simulink model "HyQ2Max_Leg_2Dof_ForAc1"  (Simulink 7.0)
settings: Solver=ode15s  StartTime=0.0  StopTime=6.0  MaxStep=1e-2  RelTol=1e-3
values from neighbouring files (symbols this model uses):
  L_LegInertiab_CAD = [ ... (first row only)    [HyQ2Max_CAD_For_SimMechanics_LF_RF.m]
  L_LegMb = 1.406    [HyQ2Max_CAD_For_SimMechanics_LF_RF.m]
  U_LegInertia_CAD = [0.010196 0.002320 0.000141 ... (first row only)    [HyQ2Max_CAD_For_SimMechanics_LF_RF.m]
  U_LegM = 4.95    [HyQ2Max_CAD_For_SimMechanics_LF_RF.m]
libraries: mblibv1 x24, fl_lib x6, nesl_utility x4, simulink_extras x2
settings Model: Creator=Gustavo  LastModifiedBy=Gustavo
settings SolverCC: SolverResetMethod=Robust
settings DebuggingCC: SaveWithParameterizedLinksMsg=none  SignalResolutionControl=TryResolveAllWithWarning  MultiTaskDSMMsg=warning  MultiTaskCondExecSysMsg=none
settings RTWCC: IncludeERTFirstTime=on
settings GRTTargetCC: TargetFcnLib=ansi_tfl_tmw.mat
settings SimMechanicsCC: VisOnUpdateDiagram=on  VisDuringSimulation=on

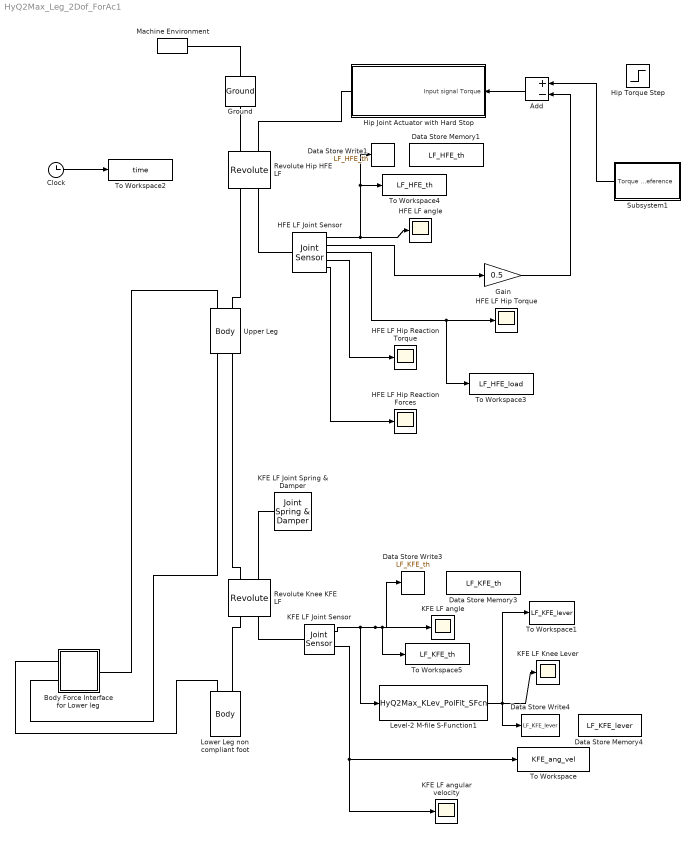
== system HyQ2Max_Leg_2Dof_ForAc1 ==
  Add : Sum  Orientation=left  Inputs=+-  OutDataType=sfix(16)  OutScaling=2^-10
  Body Force Interface for Lower leg : Subsystem
  Clock : Clock
      settings: Decimation=10
  Data Store Memory1 : DataStoreMemory  DataStoreName=LF_HFE_th  ReadBeforeWriteMsg=warning  WriteAfterWriteMsg=warning  WriteAfterReadMsg=warning  OutDataType=sfix(16)  OutScaling=2^0
  Data Store Memory3 : DataStoreMemory  DataStoreName=LF_KFE_th  ReadBeforeWriteMsg=warning  WriteAfterWriteMsg=warning  WriteAfterReadMsg=warning  OutDataType=sfix(16)  OutScaling=2^0
  Data Store Memory4 : DataStoreMemory  DataStoreName=LF_KFE_lever  ReadBeforeWriteMsg=warning  WriteAfterWriteMsg=warning  WriteAfterReadMsg=warning  OutDataType=sfix(16)  OutScaling=2^0
  Data Store Write1 : DataStoreWrite  DataStoreName=LF_HFE_th  SampleTime=-1
  Data Store Write3 : DataStoreWrite  DataStoreName=LF_KFE_th  SampleTime=-1
  Data Store Write4 : DataStoreWrite  DataStoreName=LF_KFE_lever  SampleTime=-1
  Gain : Gain  Gain=0.5  ParameterDataType=sfix(16)  ParameterScaling=2^0  OutDataType=sfix(16)  OutScaling=2^0
  Ground : mblibv1/Bodies/Ground  Orientation=down  DialogController=MECH.DynMechDlgSource  SystemSampleTime=-1  LeftPortType=env  RightPortType=workingframe  PhysicalDomain=Mechanical  DialogClass=GroundBlock  CoordPosition=[0 0 0]  CoordPositionUnits=m  StateVectorMgrId=-1  MachineId=[0 0]  ShowEnvPort=on
  HFE LF Joint Sensor : mblibv1/Sensors &  Actuators/Joint Sensor  DialogController=MECH.DynMechDlgSource  SystemSampleTime=-1  PhysicalDomain=Mechanical  PortType=blob  Muxed=off  Pose=off  Angle=on  AngleUnits=rad  ArcVelocity=on  ArcVelocityUnits=rad/s  ArcAcceleration=off  ArcAccelerationUnits=rad/s^2  CoordPosition=on  CoordPositionUnits=m  Velocity=off  VelocityUnits=m/s  Acceleration=off  AccelerationUnits=m/s^2  Quaternion=on  QuaternionDT=off  QuaternionDDT=off  QuaternionUnits=off  OutputVector=[ 1 ]  ActiveIO=on  Width=9  DialogClass=MechanicalSensorBlock  Primitive=R1  Force=off  ForceUnits=N  Torque=on  TorqueUnits=N*m  ReferenceFrame=Absolute (INERTIAL)  ReactionSensedSide=Base  ReactionReferenceFrame=Absolute (World)  ReactionForce=on  ReactionForceUnits=N  ReactionMoment=on  ReactionMomentUnits=N*m
  HFE LF Hip Reaction Forces : Scope
      settings: YMin=-40  YMax=40  SaveName=ScopeData6
  HFE LF Hip Reaction Torque : Scope
      settings: YMin=-0.4  YMax=0.3  SaveName=ScopeData7
  HFE LF Hip Torque : Scope
      settings: TimeRange=6  YMin=-10000  YMax=10000  SaveName=ScopeData4
  HFE LF angle : Scope
      settings: YMin=-0.1  YMax=1
  Hip Joint Actuator with Hard Stop : Subsystem  Orientation=left
  Hip Torque Step : Step  Orientation=left  After=5  SampleTime=0
  KFE LF Joint Sensor : mblibv1/Sensors &  Actuators/Joint Sensor  DialogController=MECH.DynMechDlgSource  SystemSampleTime=-1  PhysicalDomain=Mechanical  PortType=blob  Muxed=off  Pose=off  Angle=on  AngleUnits=rad  ArcVelocity=on  ArcVelocityUnits=rad/s  ArcAcceleration=off  ArcAccelerationUnits=rad/s^2  CoordPosition=on  CoordPositionUnits=m  Velocity=off  VelocityUnits=m/s  Acceleration=off  AccelerationUnits=m/s^2  Quaternion=on  QuaternionDT=off  QuaternionDDT=off  QuaternionUnits=off  OutputVector=[ 1 ]  ActiveIO=on  Width=2  DialogClass=MechanicalSensorBlock  Primitive=R1  Force=off  ForceUnits=N  Torque=off  TorqueUnits=N*m  ReferenceFrame=Absolute (INERTIAL)  ReactionSensedSide=Base  ReactionReferenceFrame=Absolute (World)  ReactionForce=off  ReactionForceUnits=N  ReactionMoment=off  ReactionMomentUnits=N*m
  KFE LF Joint Spring & Damper : mblibv1/Force  Elements/Joint Spring & Damper  DialogController=MECH.DynMechDlgSource  SystemSampleTime=-1  DialogClass=JointSpringDamper  JFEParameters=P1$false$0$0$0$m$m/s$N$deg$deg/s$N*m#P2$false$0$0$0$m$m/s$N$deg$deg/s$N*m#P3$false$0$0$0$m$m/s$N$deg$deg/s$N*m#R1$true$0$0.5$0$m$m/s$N$rad$rad/s$N*m#R2$false$0$0$0$m$m/s$N$deg$deg/s$N*m#R3$false$0$0$0$m$m/s$N$deg$deg/s$N*m#S$false$0$0$0$m$m/s$N$deg$deg/s$N*m
  KFE LF Knee Lever : Scope
      settings: YMin=0.005  YMax=0.04  SaveName=ScopeData9
  KFE LF angle : Scope
      settings: YMin=-2.5  YMax=0  SaveName=ScopeData8
  KFE LF angular velocity : Scope
      settings: YMin=-3.5  YMax=3.5
  Level-2 M-file S-Function1 : M-S-Function  FunctionName=HyQ2Max_KLev_PolFit_SFcn
  Lower Leg non compliant foot : mblibv1/Bodies/Body  Orientation=down  DialogController=MECH.DynMechDlgSource  PhysicalDomain=mechanical  SubClassName=Unknown  LeftPortType=workingframe  RightPortType=workingframe  LConnTagsString=CS3|CS1  RConnTagsString=CS2  DialogClass=MechanicalBodyBlock  Mass=L_LegMb  MassUnits=kg  InertiaUnits=kg*m^2  Inertia=L_LegInertiab_CAD  Shape=Cylinder  ShapeDims=[1 1]  ShapeUnits=m  ShapeUse=false  Density=1  DensityUnits=kg/m^3  DensityUse=false  CG=Left$CG$L_LegCogb_CAD$CS1$CS1$m$[-90 180 0]$Euler Z-X-Z$deg$World$false  WorkingFrames="Left$CS3$[0.0262 0.0216 0]$CS1$CS1$m$[-90 180 0]$Euler Z-X-Z$deg$World$true#Left$CS1$[0 0  0]$Adjoining$Adjoining$m$[-90 180 0]$Euler Z-X-Z$deg$World$true#Right$CS2$[0.38009 0 0]$CS1$CS1$m$[-90 180 0]$Euler Z-X-Z$deg$World$true"  CGPos=L_LegCogb_CAD  CGRot=[-90 180 0]  CS0Pos=[]  CS0Rot=[]  CS1Pos="[0 0  0]"  CS1Rot=[-90 180 0]  CS2Pos=[0.38009 0 0]  CS2Rot=[-90 180 0]  CS3Pos=[0.0262 0.0216 0]  CS3Rot=[-90 180 0]  CS4Pos=[]  CS4Rot=[]  CS5Pos=[]  CS5Rot=[]  CS6Pos=[]  CS6Rot=[]  CS7Pos=[]  CS7Rot=[]  CS8Pos=[]  CS8Rot=[]  CS9Pos=[]  CS9Rot=[]  CS10Pos=[]  CS10Rot=[]  CS11Pos=[]  CS11Rot=[]  CS12Pos=[]  CS12Rot=[]  CS13Pos=[]  CS13Rot=[]  CS14Pos=[]  CS14Rot=[]  CS15Pos=[]  CS15Rot=[]  CS16Pos=[]  CS16Rot=[]  CS17Pos=[]  CS17Rot=[]  CS18Pos=[]  CS18Rot=[]  CS19Pos=[]  CS19Rot=[]  CS20Pos=[]  CS20Rot=[]
  Machine Environment : mblibv1/Bodies/Machine Environment  Tag=Factory ground  DialogController=MECH.DialogSource  SystemSampleTime=-1  PortType=env  PhysicalDomain=Mechanical  DialogTemplateClass=MECH.MachineEnvironment  SyncWhenCopied=off  Gravity=[0 -9.81 0]  GravityUnits=m/s^2  GravityAsSignal=off  Dimensionality=Auto-detect  AnalysisType=Forward dynamics  LinearAssemblyTolerance=1e-3  LinearAssemblyToleranceUnits=m  AngularAssemblyTolerance=1e-3  AngularAssemblyToleranceUnits=rad  ConstraintSolverType=Stabilizing  ConstraintRelTolerance=1e-4  ConstraintAbsTolerance=1e-4  UseRobustSingularityHandling=off  RedundancyAnalysisToleranceType=Automatically select tolerance  RedundancyAnalysisTolerance=1e-14  StatePerturbationType=Fixed  PerturbationSize=1e-5  VisualizeMachine=on
  Revolute Hip HFE LF : mblibv1/Joints/Revolute  Orientation=down  DialogController=MECH.DynMechDlgSource  PhysicalDomain=mechanical  SubClassName=Unknown  LeftPortType=blob  RightPortType=blob  LConnTagsString=__newl0|SA1  RConnTagsString=__newr0|SA1  NumSAPorts=2  CutJoint=off  MarkAsCut=off  Primitives=revolute  PrimitiveProps=R1$World$[0 0 -1]$revolute  DialogClass=JointBlock  R1Axis=[0 0 -1]
  Revolute Knee KFE LF : mblibv1/Joints/Revolute  Orientation=down  DialogController=MECH.DynMechDlgSource  PhysicalDomain=mechanical  SubClassName=Unknown  LeftPortType=blob  RightPortType=blob  LConnTagsString=__newl0|SA1  RConnTagsString=__newr0|SA1  NumSAPorts=2  CutJoint=off  MarkAsCut=off  Primitives=revolute  PrimitiveProps=R1$World$[0 0 -1]$revolute  DialogClass=JointBlock  R1Axis=[0 0 -1]
  Subsystem1 : Subsystem  Orientation=left
  To Workspace : ToWorkspace  VariableName=KFE_ang_vel  SampleTime=-1  SaveFormat=Array
  To Workspace1 : ToWorkspace  VariableName=LF_KFE_lever  SampleTime=-1  SaveFormat=Array
  To Workspace2 : ToWorkspace  VariableName=time  SampleTime=-1  SaveFormat=Array
  To Workspace3 : ToWorkspace  VariableName=LF_HFE_load  SampleTime=-1  SaveFormat=Array
  To Workspace4 : ToWorkspace  VariableName=LF_HFE_th  SampleTime=-1  SaveFormat=Array
  To Workspace5 : ToWorkspace  VariableName=LF_KFE_th  SampleTime=-1  SaveFormat=Array
  Upper Leg : mblibv1/Bodies/Body  Orientation=down  DialogController=MECH.DynMechDlgSource  PhysicalDomain=mechanical  SubClassName=Unknown  LeftPortType=workingframe  RightPortType=workingframe  LConnTagsString=CS4|CS1  RConnTagsString=CS3|CS2  DialogClass=MechanicalBodyBlock  Mass=U_LegM  MassUnits=kg  InertiaUnits=kg*m^2  Inertia=U_LegInertia_CAD  Shape=Cylinder  ShapeDims=[1 1]  ShapeUnits=m  ShapeUse=false  Density=1  DensityUnits=kg/m^3  DensityUse=false  CG=Left$CG$U_LegCog_CAD$CS1$CS1$m$[-90 180 0]$Euler Z-X-Z$deg$WORLD$false  WorkingFrames="Left$CS4$[-.041 -.005 0]$CS1$CS1$m$[-90 180 0]$Euler Z-X-Z$deg$WORLD$true#Right$CS3$[.32  .023 0]$CS1$CS1$m$[-90 180 0]$Euler Z-X-Z$deg$WORLD$true#Left$CS1$[0 0 0]$World$World$m$[-90 180 0]$Euler Z-X-Z$deg$World$true#Right$CS2$[.36 0 0]$CS1$CS1$m$[-90 180 0]$Euler Z-X-Z$deg$World$true"  CGPos=U_LegCog_CAD  CGRot=[-90 180 0]  CS0Pos=[]  CS0Rot=[]  CS1Pos=[0 0 0]  CS1Rot=[-90 180 0]  CS2Pos=[.36 0 0]  CS2Rot=[-90 180 0]  CS3Pos="[.32  .023 0]"  CS3Rot=[-90 180 0]  CS4Pos=[-.041 -.005 0]  CS4Rot=[-90 180 0]  CS5Pos=[]  CS5Rot=[]  CS6Pos=[]  CS6Rot=[]  CS7Pos=[]  CS7Rot=[]  CS8Pos=[]  CS8Rot=[]  CS9Pos=[]  CS9Rot=[]  CS10Pos=[]  CS10Rot=[]  CS11Pos=[]  CS11Rot=[]  CS12Pos=[]  CS12Rot=[]  CS13Pos=[]  CS13Rot=[]  CS14Pos=[]  CS14Rot=[]  CS15Pos=[]  CS15Rot=[]  CS16Pos=[]  CS16Rot=[]  CS17Pos=[]  CS17Rot=[]  CS18Pos=[]  CS18Rot=[]  CS19Pos=[]  CS19Rot=[]  CS20Pos=[]  CS20Rot=[]
  wires:
  HFE LF Joint Sensor/1 -> HFE LF angle/1, To Workspace4/1, Data Store Write1/1
  KFE LF Joint Sensor/1 -> Level-2 M-file S-Function1/1, KFE LF angle/1, To Workspace5/1, Data Store Write3/1
  Level-2 M-file S-Function1/1 -> KFE LF Knee Lever/1, To Workspace1/1, Data Store Write4/1
  Gain/1 -> Add/2
  Add/1 -> Hip Joint Actuator with Hard Stop/1(Input signal Torque)
  HFE LF Joint Sensor/5 -> HFE LF Hip Reaction Forces/1
  HFE LF Joint Sensor/4 -> HFE LF Hip Reaction Torque/1
  HFE LF Joint Sensor/3 -> HFE LF Hip Torque/1, To Workspace3/1
  HFE LF Joint Sensor/2 -> Gain/1
  KFE LF Joint Sensor/2 -> KFE LF angular velocity/1, To Workspace/1
  Clock/1 -> To Workspace2/1
  Subsystem1/1(Torque Reference) -> Add/1
  connections:
  HFE LF Joint Sensor/LConn1 -- Revolute Hip HFE LF/RConn2
  Machine Environment/RConn1 -- Ground/LConn1
  Ground/RConn1 -- Revolute Hip HFE LF/LConn1
  Revolute Hip HFE LF/RConn1 -- Upper Leg/LConn2
  Upper Leg/RConn2 -- Revolute Knee KFE LF/LConn1
  KFE LF Joint Sensor/LConn1 -- Revolute Knee KFE LF/RConn2
  Lower Leg non compliant foot/LConn2 -- Revolute Knee KFE LF/RConn1
  Lower Leg non compliant foot/LConn1 -- Body Force Interface for Lower leg/LConn1
  Revolute Knee KFE LF/LConn2 -- KFE LF Joint Spring & Damper/LConn1
  Hip Joint Actuator with Hard Stop/RConn1 -- Revolute Hip HFE LF/LConn2
  Body Force Interface for Lower leg/RConn1 -- Upper Leg/LConn1
  Upper Leg/RConn1 -- Body Force Interface for Lower leg/LConn2

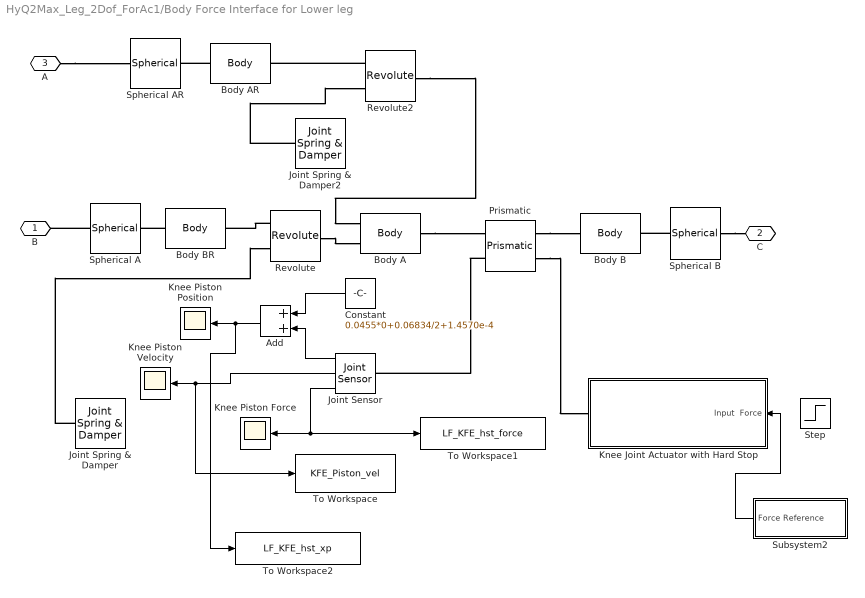
== system HyQ2Max_Leg_2Dof_ForAc1/Body Force Interface for Lower leg ==
  Add : Sum  Orientation=left  OutDataType=sfix(16)  OutScaling=2^-10
  Body A : mblibv1/Bodies/Body  DialogController=MECH.DynMechDlgSource  PhysicalDomain=mechanical  SubClassName=Unknown  LeftPortType=workingframe  RightPortType=workingframe  LConnTagsString=CS3|CS1  RConnTagsString=CS2  DialogClass=MechanicalBodyBlock  Mass=0.09  MassUnits=kg  InertiaUnits=kg*m^2  Inertia=eye(3)*1e-4  Shape=Cylinder  ShapeDims=[1 1]  ShapeUnits=m  ShapeUse=false  Density=1  DensityUnits=kg/m^3  DensityUse=false  CG=Left$CG$[-.3935857/2 0 0]$CS1$CS1$m$[0 0 0]$Euler X-Y-Z$deg$CS1$false  WorkingFrames=Left$CS3$[0 0 0]$Adjoining$Adjoining$m$[0 0 0]$Euler X-Y-Z$deg$Adjoining$true#Left$CS1$[0 0 0]$Adjoining$Adjoining$m$[0 0 -55.1441]$Euler X-Y-Z$deg$Adjoining$true#Right$CS2$[-.3935857 0 0]$CS1$CS1$m$[0 0 0]$Euler X-Y-Z$deg$CS1$true  CGPos=[-.3935857/2 0 0]  CGRot=[0 0 0]  CS0Pos=[]  CS0Rot=[]  CS1Pos=[0 0 0]  CS1Rot=[0 0 -55.1441]  CS2Pos=[-.3935857 0 0]  CS2Rot=[0 0 0]  CS3Pos=[0 0 0]  CS3Rot=[0 0 0]  CS4Pos=[]  CS4Rot=[]  CS5Pos=[]  CS5Rot=[]  CS6Pos=[]  CS6Rot=[]  CS7Pos=[]  CS7Rot=[]  CS8Pos=[]  CS8Rot=[]  CS9Pos=[]  CS9Rot=[]  CS10Pos=[]  CS10Rot=[]  CS11Pos=[]  CS11Rot=[]  CS12Pos=[]  CS12Rot=[]  CS13Pos=[]  CS13Rot=[]  CS14Pos=[]  CS14Rot=[]  CS15Pos=[]  CS15Rot=[]  CS16Pos=[]  CS16Rot=[]  CS17Pos=[]  CS17Rot=[]  CS18Pos=[]  CS18Rot=[]  CS19Pos=[]  CS19Rot=[]  CS20Pos=[]  CS20Rot=[]
  Body AR : mblibv1/Bodies/Body  DialogController=MECH.DynMechDlgSource  PhysicalDomain=mechanical  SubClassName=Unknown  LeftPortType=workingframe  RightPortType=workingframe  LConnTagsString=CS1  RConnTagsString=CS2  DialogClass=MechanicalBodyBlock  Mass=0.01  MassUnits=kg  InertiaUnits=kg*m^2  Inertia=eye(3)*1e-3  Shape=Cylinder  ShapeDims=[1 1]  ShapeUnits=m  ShapeUse=false  Density=1  DensityUnits=kg/m^3  DensityUse=false  CG=Left$CG$[.056/2 0 0]$CS1$CS1$m$[0 0 0]$Euler X-Y-Z$deg$CS1$false  WorkingFrames=Left$CS1$[0 0 0]$Adjoining$Adjoining$m$[0 0 -52.3270]$Euler X-Y-Z$deg$Adjoining$true#Right$CS2$[.056 0 0]$CS1$CS1$m$[0 0 0]$Euler X-Y-Z$deg$CS1$true  CGPos=[.056/2 0 0]  CGRot=[0 0 0]  CS0Pos=[]  CS0Rot=[]  CS1Pos=[0 0 0]  CS1Rot=[0 0 -52.3270]  CS2Pos=[.056 0 0]  CS2Rot=[0 0 0]  CS3Pos=[]  CS3Rot=[]  CS4Pos=[]  CS4Rot=[]  CS5Pos=[]  CS5Rot=[]  CS6Pos=[]  CS6Rot=[]  CS7Pos=[]  CS7Rot=[]  CS8Pos=[]  CS8Rot=[]  CS9Pos=[]  CS9Rot=[]  CS10Pos=[]  CS10Rot=[]  CS11Pos=[]  CS11Rot=[]  CS12Pos=[]  CS12Rot=[]  CS13Pos=[]  CS13Rot=[]  CS14Pos=[]  CS14Rot=[]  CS15Pos=[]  CS15Rot=[]  CS16Pos=[]  CS16Rot=[]  CS17Pos=[]  CS17Rot=[]  CS18Pos=[]  CS18Rot=[]  CS19Pos=[]  CS19Rot=[]  CS20Pos=[]  CS20Rot=[]
  Body B : mblibv1/Bodies/Body  DialogController=MECH.DynMechDlgSource  PhysicalDomain=mechanical  SubClassName=Unknown  LeftPortType=workingframe  RightPortType=workingframe  LConnTagsString=CS1  RConnTagsString=CS2  DialogClass=MechanicalBodyBlock  Mass=0.09  MassUnits=kg  InertiaUnits=kg*m^2  Inertia=eye(3)*1e-4  Shape=Cylinder  ShapeDims=[1 1]  ShapeUnits=m  ShapeUse=false  Density=1  DensityUnits=kg/m^3  DensityUse=false  CG=Left$CG$[-.3935857/2 0 0]$CS1$CS1$m$[0 0 0]$Euler X-Y-Z$deg$CS1$false  WorkingFrames=Left$CS1$[.3935857 0 0]$Adjoining$Adjoining$m$[0 0 0]$Euler X-Y-Z$deg$Adjoining$true#Right$CS2$[-.3935857 0 0]$CS1$CS1$m$[0 0 0]$Euler X-Y-Z$deg$CS1$true  CGPos=[-.3935857/2 0 0]  CGRot=[0 0 0]  CS0Pos=[]  CS0Rot=[]  CS1Pos=[.3935857 0 0]  CS1Rot=[0 0 0]  CS2Pos=[-.3935857 0 0]  CS2Rot=[0 0 0]  CS3Pos=[]  CS3Rot=[]  CS4Pos=[]  CS4Rot=[]  CS5Pos=[]  CS5Rot=[]  CS6Pos=[]  CS6Rot=[]  CS7Pos=[]  CS7Rot=[]  CS8Pos=[]  CS8Rot=[]  CS9Pos=[]  CS9Rot=[]  CS10Pos=[]  CS10Rot=[]  CS11Pos=[]  CS11Rot=[]  CS12Pos=[]  CS12Rot=[]  CS13Pos=[]  CS13Rot=[]  CS14Pos=[]  CS14Rot=[]  CS15Pos=[]  CS15Rot=[]  CS16Pos=[]  CS16Rot=[]  CS17Pos=[]  CS17Rot=[]  CS18Pos=[]  CS18Rot=[]  CS19Pos=[]  CS19Rot=[]  CS20Pos=[]  CS20Rot=[]
  Body BR : mblibv1/Bodies/Body  DialogController=MECH.DynMechDlgSource  PhysicalDomain=mechanical  SubClassName=Unknown  LeftPortType=workingframe  RightPortType=workingframe  LConnTagsString=CS1  RConnTagsString=CS2  DialogClass=MechanicalBodyBlock  Mass=0.01  MassUnits=kg  InertiaUnits=kg*m^2  Inertia=eye(3)*1e-3  Shape=Cylinder  ShapeDims=[1 1]  ShapeUnits=m  ShapeUse=false  Density=1  DensityUnits=kg/m^3  DensityUse=false  CG=Left$CG$[-.056/2 0 0]$CS1$CS1$m$[0 0 0]$Euler X-Y-Z$deg$CS1$false  WorkingFrames=Left$CS1$[0 0 0]$Adjoining$Adjoining$m$[0 0 52.5477]$Euler X-Y-Z$deg$Adjoining$true#Right$CS2$[-.056 0 0]$CS1$CS1$m$[0 0 0]$Euler X-Y-Z$deg$CS1$true  CGPos=[-.056/2 0 0]  CGRot=[0 0 0]  CS0Pos=[]  CS0Rot=[]  CS1Pos=[0 0 0]  CS1Rot=[0 0 52.5477]  CS2Pos=[-.056 0 0]  CS2Rot=[0 0 0]  CS3Pos=[]  CS3Rot=[]  CS4Pos=[]  CS4Rot=[]  CS5Pos=[]  CS5Rot=[]  CS6Pos=[]  CS6Rot=[]  CS7Pos=[]  CS7Rot=[]  CS8Pos=[]  CS8Rot=[]  CS9Pos=[]  CS9Rot=[]  CS10Pos=[]  CS10Rot=[]  CS11Pos=[]  CS11Rot=[]  CS12Pos=[]  CS12Rot=[]  CS13Pos=[]  CS13Rot=[]  CS14Pos=[]  CS14Rot=[]  CS15Pos=[]  CS15Rot=[]  CS16Pos=[]  CS16Rot=[]  CS17Pos=[]  CS17Rot=[]  CS18Pos=[]  CS18Rot=[]  CS19Pos=[]  CS19Rot=[]  CS20Pos=[]  CS20Rot=[]
  Constant : Constant  Orientation=left  Value=0.0455*0+0.06834/2+1.4570e-4  OutDataType=sfix(16)  OutScaling=2^0
  Joint Spring & Damper : mblibv1/Force  Elements/Joint Spring & Damper  DialogController=MECH.DynMechDlgSource  SystemSampleTime=-1  DialogClass=JointSpringDamper  JFEParameters=P1$false$0$0$0$m$m/s$N$deg$deg/s$N*m#P2$false$0$0$0$m$m/s$N$deg$deg/s$N*m#P3$false$0$0$0$m$m/s$N$deg$deg/s$N*m#R1$false$0$0.5$0$m$m/s$N$rad$rad/s$N*m#R2$false$0$0$0$m$m/s$N$deg$deg/s$N*m#R3$false$0$0$0$m$m/s$N$deg$deg/s$N*m#S$false$0$0$0$m$m/s$N$deg$deg/s$N*m
  Joint Spring & Damper2 : mblibv1/Force  Elements/Joint Spring & Damper  DialogController=MECH.DynMechDlgSource  SystemSampleTime=-1  DialogClass=JointSpringDamper  JFEParameters=P1$false$0$0$0$m$m/s$N$deg$deg/s$N*m#P2$false$0$0$0$m$m/s$N$deg$deg/s$N*m#P3$false$0$0$0$m$m/s$N$deg$deg/s$N*m#R1$false$0$0.5$0$m$m/s$N$rad$rad/s$N*m#R2$false$0$0$0$m$m/s$N$deg$deg/s$N*m#R3$false$0$0$0$m$m/s$N$deg$deg/s$N*m#S$false$0$0$0$m$m/s$N$deg$deg/s$N*m
  Joint Sensor : mblibv1/Sensors &  Actuators/Joint Sensor  Orientation=left  DialogController=MECH.DynMechDlgSource  SystemSampleTime=-1  PhysicalDomain=Mechanical  PortType=blob  Muxed=off  Pose=off  Angle=on  AngleUnits=deg  ArcVelocity=off  ArcVelocityUnits=deg/s  ArcAcceleration=off  ArcAccelerationUnits=deg/s^2  CoordPosition=on  CoordPositionUnits=m  Velocity=on  VelocityUnits=m/s  Acceleration=off  AccelerationUnits=m/s^2  Quaternion=on  QuaternionDT=off  QuaternionDDT=off  QuaternionUnits=off  OutputVector=[1]  ActiveIO=on  Width=3  DialogClass=MechanicalSensorBlock  Primitive=P1  Force=on  ForceUnits=N  Torque=off  TorqueUnits=N*m  ReferenceFrame=Absolute (World)  ReactionSensedSide=Base  ReactionReferenceFrame=Absolute (World)  ReactionForce=off  ReactionForceUnits=N  ReactionMoment=off  ReactionMomentUnits=N*m
  Knee Joint Actuator with Hard Stop : Subsystem  Orientation=left
  Knee Piston Force : Scope
      settings: TimeRange=6  YMin=-250000  YMax=175000  SaveName=ScopeData2
  Knee Piston Position : Scope
      settings: YMin=-0.035  YMax=0.035  SaveName=ScopeData3
  Knee Piston Velocity : Scope
      settings: YMin=-0.035  YMax=0.035  SaveName=ScopeData5
  Prismatic : mblibv1/Joints/Prismatic  Orientation=left  DialogController=MECH.DynMechDlgSource  PhysicalDomain=mechanical  SubClassName=Unknown  LeftPortType=blob  RightPortType=blob  LConnTagsString=__newl0|SA1  RConnTagsString=__newr0|SA1  NumSAPorts=2  CutJoint=off  MarkAsCut=off  Primitives=prismatic  PrimitiveProps=P1$Base$[1 0 0]$prismatic  DialogClass=JointBlock  P1Axis=[1 0 0]
  Revolute : mblibv1/Joints/Revolute  DialogController=MECH.DynMechDlgSource  PhysicalDomain=mechanical  SubClassName=Unknown  LeftPortType=blob  RightPortType=blob  LConnTagsString=__newl0|SA1  RConnTagsString=__newr0  NumSAPorts=1  CutJoint=off  MarkAsCut=off  Primitives=prismatic  PrimitiveProps=R1$Follower$[0 0 1]$revolute  DialogClass=JointBlock  R1Axis=[0 0 1]
  Revolute2 : mblibv1/Joints/Revolute  DialogController=MECH.DynMechDlgSource  PhysicalDomain=mechanical  SubClassName=Unknown  LeftPortType=blob  RightPortType=blob  LConnTagsString=__newl0|SA1  RConnTagsString=__newr0  NumSAPorts=1  CutJoint=off  MarkAsCut=off  Primitives=prismatic  PrimitiveProps=R1$Follower$[0 0 1]$revolute  DialogClass=JointBlock  R1Axis=[0 0 1]
  "Spherical A " : mblibv1/Joints/Spherical  DialogController=MECH.DynMechDlgSource  PhysicalDomain=mechanical  SubClassName=Unknown  LeftPortType=blob  RightPortType=blob  LConnTagsString=__newl0  RConnTagsString=__newr0  NumSAPorts=0  CutJoint=off  MarkAsCut=off  Primitives=spherical  PrimitiveProps=S$WORLD$[0 0 0]$spherical  DialogClass=JointBlock  SAxis=[0 0 0]
  Spherical AR : mblibv1/Joints/Spherical  DialogController=MECH.DynMechDlgSource  PhysicalDomain=mechanical  SubClassName=Unknown  LeftPortType=blob  RightPortType=blob  LConnTagsString=__newl0  RConnTagsString=__newr0  NumSAPorts=0  CutJoint=off  MarkAsCut=off  Primitives=spherical  PrimitiveProps=S$WORLD$[0 0 0]$spherical  DialogClass=JointBlock  SAxis=[0 0 0]
  Spherical B : mblibv1/Joints/Spherical  DialogController=MECH.DynMechDlgSource  PhysicalDomain=mechanical  SubClassName=Unknown  LeftPortType=blob  RightPortType=blob  LConnTagsString=__newl0  RConnTagsString=__newr0  NumSAPorts=0  CutJoint=off  MarkAsCut=off  Primitives=spherical  PrimitiveProps=S$World$[0 0 0]$spherical  DialogClass=JointBlock  SAxis=[0 0 0]
  Step : Step  Orientation=left  Time=2  After=-20*1.8  SampleTime=0
  Subsystem2 : Subsystem  Orientation=left
  To Workspace : ToWorkspace  VariableName=KFE_Piston_vel  SampleTime=-1  SaveFormat=Array
  To Workspace1 : ToWorkspace  VariableName=LF_KFE_hst_force  SampleTime=-1  SaveFormat=Array
  To Workspace2 : ToWorkspace  VariableName=LF_KFE_hst_xp  SampleTime=-1  SaveFormat=Array
  B : PMIOPort  Port=1  Side=Left
  C : PMIOPort  Orientation=left  Port=2  Side=Right
  A : PMIOPort  Port=3  Side=Left
  wires:
  Constant/1 -> Add/1
  Add/1 -> Knee Piston Position/1, To Workspace2/1
  Joint Sensor/1 -> Add/2
  Joint Sensor/3 -> Knee Piston Force/1, To Workspace1/1
  Joint Sensor/2 -> Knee Piston Velocity/1, To Workspace/1
  Subsystem2/1(Force Reference) -> Knee Joint Actuator with Hard Stop/1(Input  Force)
  connections:
  Body A/RConn1 -- Prismatic/RConn1
  Prismatic/LConn1 -- Body B/LConn1
  Prismatic/LConn2 -- Knee Joint Actuator with Hard Stop/RConn1
  Spherical B/RConn1 -- C/RConn1
  Spherical B/LConn1 -- Body B/RConn1
  Prismatic/RConn2 -- Joint Sensor/LConn1
  "Spherical A "/LConn1 -- B/RConn1
  Body BR/LConn1 -- "Spherical A "/RConn1
  Revolute/RConn1 -- Body A/LConn2
  Revolute/LConn1 -- Body BR/RConn1
  Joint Spring & Damper/LConn1 -- Revolute/LConn2
  Body AR/LConn1 -- Spherical AR/RConn1
  Revolute2/RConn1 -- Body A/LConn1
  Revolute2/LConn1 -- Body AR/RConn1
  Joint Spring & Damper2/LConn1 -- Revolute2/LConn2
  A/RConn1 -- Spherical AR/LConn1

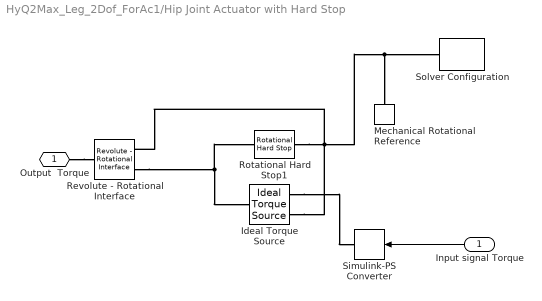
== system HyQ2Max_Leg_2Dof_ForAc1/Hip Joint Actuator with Hard Stop ==
  Input signal Torque : Inport  Orientation=left
  Ideal Torque Source : fl_lib/Mechanical/Mechanical Sensors and Sources/Ideal Torque Source  DialogController=NetworkEngine.DynNeDlgSource  SystemSampleTime=-1  torque_Log=off  rel_velocity_Log=off  power_Log=off  LocalVarNames=|torque|rel_velocity|power  LocalVarDescs=|Torque (N*m)|Relative velocity (rad/s)|Power generated by the source (W)  LocalVarLogging=[0 0 0]
  Mechanical Rotational Reference : fl_lib/Mechanical/Rotational Elements/Mechanical Rotational Reference  Orientation=down  DialogController=NetworkEngine.DynNeDlgSource  SystemSampleTime=-1  LocalVarLogging=[]
  Revolute - Rotational Interface : mblibv1/Interface  Elements/Revolute - Rotational Interface  Orientation=left  DialogController=MECH.DynMechDlgSource  SystemSampleTime=-1  DialogClass=RevoluteRotationalInterface  Primitive=R1
  Rotational Hard Stop1 : fl_lib/Mechanical/Rotational Elements/Rotational Hard Stop  DialogController=NetworkEngine.DynNeDlgSource  SystemSampleTime=-1  upper_bnd=135/180*pi rad  lower_bnd=-135/180*pi rad  stiff_up=1e+06 N*m/rad  stiff_neg=1e+06 N*m/rad  D_up=1e4 N*m/(rad/s)  D_low=1e4 N*m/(rad/s)  contact_torque_Log=off  rel_angle_Log=off  LocalVarNames=|contact_torque|rel_angle  LocalVarDescs=|Contact torque (N*m)|Slider-case relative angle (rad)  LocalVarLogging=[0 0]
  Simulink-PS Converter : nesl_utility/Simulink-PS Converter  Orientation=left  DialogController=NetworkEngine.DynNeUtilDlgSource  SystemSampleTime=-1  PhysicalDomain=network_engine_domain  LeftPortType=input  RightPortType=output  SubClassName=ps_input  Unit=1
  Solver Configuration : nesl_utility/Solver Configuration  Orientation=left  DialogController=NetworkEngine.DynNeUtilDlgSource  SystemSampleTime=-1  PhysicalDomain=network_engine_domain  LeftPortType=input  RightPortType=generic  SubClassName=solver  ResidualTolerance=1e-9  MaxNonlinIter=12  MaxModeIter=2  DoFixedCost=on  DoDC=on  LinearAlgebra=Full  Accelerate=off
  Output  Torque : PMIOPort  Port=1  Side=Right
  wires:
  Input signal Torque/1 -> Simulink-PS Converter/1
  connections:
  Revolute - Rotational Interface/LConn2 -- Ideal Torque Source/LConn1 -- Rotational Hard Stop1/LConn1
  Ideal Torque Source/RConn1 -- Simulink-PS Converter/RConn1
  Rotational Hard Stop1/RConn1 -- Solver Configuration/RConn1 -- Mechanical Rotational Reference/LConn1 -- Ideal Torque Source/RConn2 -- Revolute - Rotational Interface/LConn1
  Output  Torque/RConn1 -- Revolute - Rotational Interface/RConn1

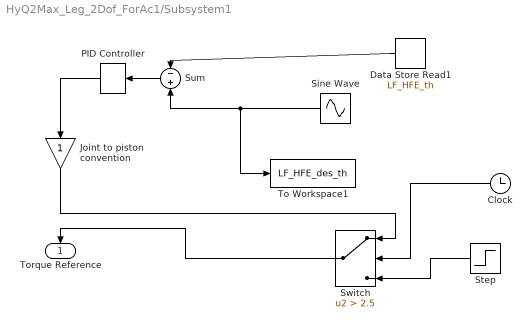
== system HyQ2Max_Leg_2Dof_ForAc1/Subsystem1 ==
  Clock : Clock
      settings: Decimation=10
  Data Store Read1 : DataStoreRead  Orientation=left  DataStoreName=LF_HFE_th  SampleTime=0
  Joint to piston    convention : Gain  Orientation=down  ParameterDataType=sfix(16)  ParameterScaling=2^0  OutDataType=sfix(16)  OutScaling=2^0
  PID Controller : simulink_extras/Additional Linear/PID Controller  Orientation=left  SystemSampleTime=-1  P=3000*3  I=0  D=600
  Sine Wave : Sin  Orientation=left  Amplitude=0.2  Bias=0.75  Frequency=8*3.1415  SampleTime=0
  Step : Step  Orientation=left  Time=2  After=0  SampleTime=0
  Sum : Sum  Orientation=left  Inputs=-|+  OutDataType=sfix(16)  OutScaling=2^0
  Switch : Switch  Orientation=left  Criteria=u2 > Threshold  Threshold=2.5  OutDataType=sfix(16)  OutScaling=2^0  ZeroCross=off
  To Workspace1 : ToWorkspace  VariableName=LF_HFE_des_th  SampleTime=-1  SaveFormat=Array
  Torque Reference : Outport  Orientation=down
  wires:
  Sum/1 -> PID Controller/1
  PID Controller/1 -> Joint to piston    convention/1
  Data Store Read1/1 -> Sum/1
  Sine Wave/1 -> To Workspace1/1, Sum/2
  Joint to piston    convention/1 -> Switch/1
  Switch/1 -> Torque Reference/1
  Step/1 -> Switch/3
  Clock/1 -> Switch/2

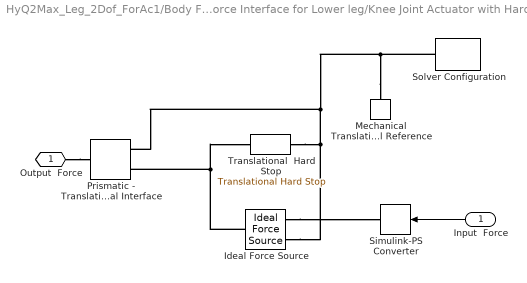
== system HyQ2Max_Leg_2Dof_ForAc1/Body Force Interface for Lower leg/Knee Joint Actuator with Hard Stop ==
  Input  Force : Inport  Orientation=left
  Ideal Force Source : fl_lib/Mechanical/Mechanical Sensors and Sources/Ideal Force Source  DialogController=NetworkEngine.DynNeDlgSource  SystemSampleTime=-1  force_Log=off  rel_velocity_Log=off  power_Log=off  LocalVarNames=|force|rel_velocity|power  LocalVarDescs=|Force (N)|Relative velocity (m/s)|Power generated by the source (W)  LocalVarLogging=[0 0 0]
  Mechanical Translational Reference : fl_lib/Mechanical/Translational Elements/Mechanical Translational Reference  Orientation=down  DialogController=NetworkEngine.DynNeDlgSource  SystemSampleTime=-1  LocalVarLogging=[]
  Prismatic - Translational Interface : mblibv1/Interface  Elements/Prismatic - Translational Interface  Orientation=left  DialogController=MECH.DynMechDlgSource  SystemSampleTime=-1  DialogClass=PrismaticTranslationalInterface  Primitive=P1
  Simulink-PS Converter : nesl_utility/Simulink-PS Converter  Orientation=left  DialogController=NetworkEngine.DynNeUtilDlgSource  SystemSampleTime=-1  PhysicalDomain=network_engine_domain  LeftPortType=input  RightPortType=output  SubClassName=ps_input  Unit=1
  Solver Configuration : nesl_utility/Solver Configuration  Orientation=left  DialogController=NetworkEngine.DynNeUtilDlgSource  SystemSampleTime=-1  PhysicalDomain=network_engine_domain  LeftPortType=input  RightPortType=generic  SubClassName=solver  ResidualTolerance=1e-9  MaxNonlinIter=12  MaxModeIter=2  DoFixedCost=on  DoDC=on  LinearAlgebra=Full  Accelerate=off
  Translational  Hard Stop : fl_lib/Mechanical/Translational Elements/Translational Hard Stop  DialogController=NetworkEngine.DynNeDlgSource  SystemSampleTime=-1  upper_bnd=-1.4570e-4 m  lower_bnd=-0.06834-1.4570e-4 m  stiff_up=1e+09 N/m  stiff_low=1e+09 N/m  D_up=1e7 N/(m/s)  D_low=1e7 N/(m/s)  contact_force_Log=off  rel_displacement_Log=off  LocalVarNames=|contact_force|rel_displacement  LocalVarDescs=|Contact force (N)|Slider-case relative displacement (m)  LocalVarLogging=[0 0]
  Output  Force : PMIOPort  Port=1  Side=Right
  wires:
  Input  Force/1 -> Simulink-PS Converter/1
  connections:
  Ideal Force Source/LConn1 -- Translational  Hard Stop/LConn1 -- Prismatic - Translational Interface/LConn2
  Ideal Force Source/RConn1 -- Simulink-PS Converter/RConn1
  Output  Force/RConn1 -- Prismatic - Translational Interface/RConn1
  Mechanical Translational Reference/LConn1 -- Solver Configuration/RConn1 -- Ideal Force Source/RConn2 -- Translational  Hard Stop/RConn1 -- Prismatic - Translational Interface/LConn1

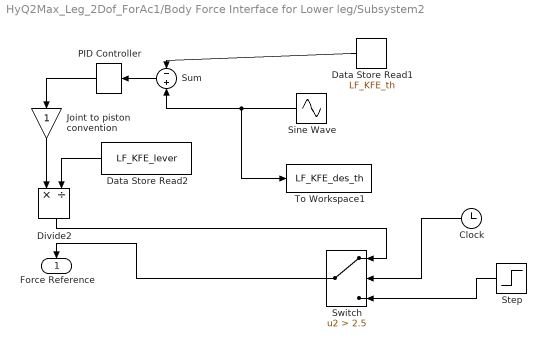
== system HyQ2Max_Leg_2Dof_ForAc1/Body Force Interface for Lower leg/Subsystem2 ==
  Clock : Clock
      settings: Decimation=10
  Data Store Read1 : DataStoreRead  Orientation=left  DataStoreName=LF_KFE_th  SampleTime=0
  Data Store Read2 : DataStoreRead  Orientation=left  DataStoreName=LF_KFE_lever  SampleTime=0
  Divide2 : Product  Orientation=down  Inputs=*/  OutDataType=sfix(16)  OutScaling=2^-10
  Joint to piston    convention : Gain  Orientation=down  ParameterDataType=sfix(16)  ParameterScaling=2^0  OutDataType=sfix(16)  OutScaling=2^0
  PID Controller : simulink_extras/Additional Linear/PID Controller  Orientation=left  SystemSampleTime=-1  P=300/1  I=0  D=6/1
  Sine Wave : Sin  Orientation=left  Amplitude=0.4  Bias=-1.5  Frequency=8*3.14  Phase=3.14  SampleTime=0
  Step : Step  Orientation=left  Time=2.0  After=0  SampleTime=0
  Sum : Sum  Orientation=left  Inputs=-|+  OutDataType=sfix(16)  OutScaling=2^0
  Switch : Switch  Orientation=left  Criteria=u2 > Threshold  Threshold=2.5  OutDataType=sfix(16)  OutScaling=2^0  ZeroCross=off
  To Workspace1 : ToWorkspace  VariableName=LF_KFE_des_th  SampleTime=-1  SaveFormat=Array
  Force Reference : Outport  Orientation=down
  wires:
  Sum/1 -> PID Controller/1
  PID Controller/1 -> Joint to piston    convention/1
  Data Store Read1/1 -> Sum/1
  Data Store Read2/1 -> Divide2/2
  Joint to piston    convention/1 -> Divide2/1
  Sine Wave/1 -> To Workspace1/1, Sum/2
  Switch/1 -> Force Reference/1
  Divide2/1 -> Switch/1
  Step/1 -> Switch/3
  Clock/1 -> Switch/2
